simulink model "sampleModel1442"  (R2023a)
settings: Solver=VariableStepAuto  StartTime=0.0  StopTime=10.0  RelTol=1e-3
libraries: hdlsllib x5
settings Model: Creator=user1  LastModifiedBy=user1

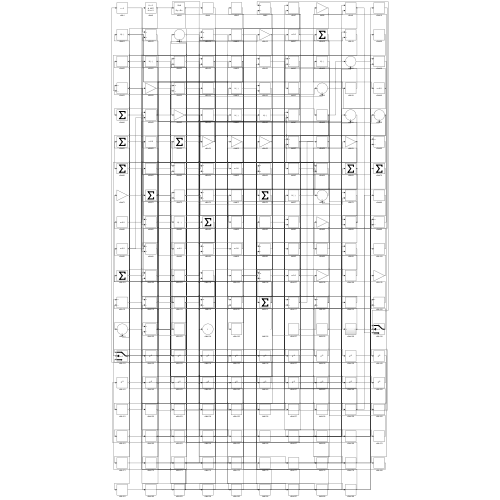
[thumbnail: Simulink's stored preview of the top-level diagram]
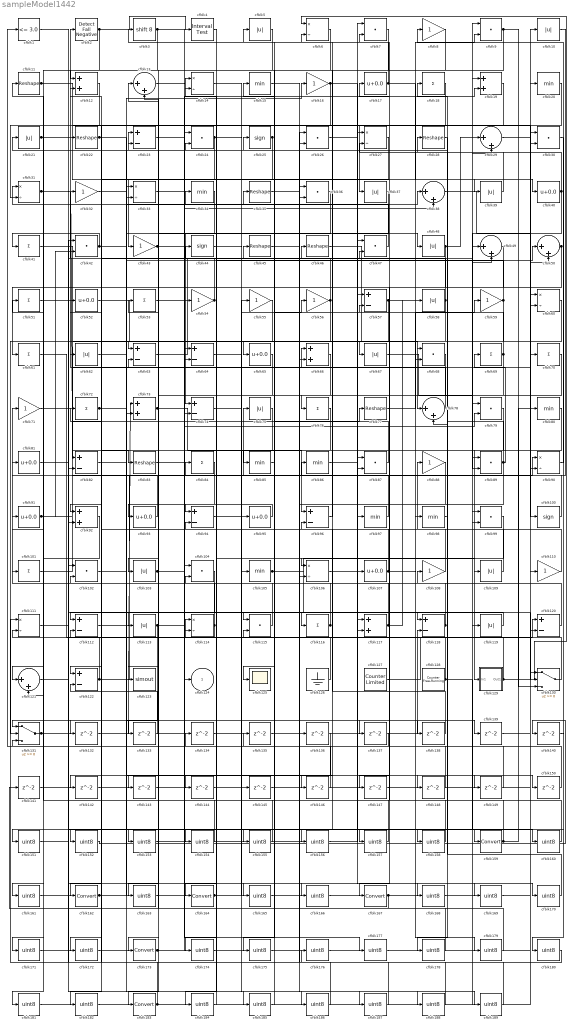
== system sampleModel1442 ==
  cfblk1 : hdlsllib/Logic and Bit Operations/Compare To Constant  relop=<=  const=3.0  OutDataTypeStr=boolean
  cfblk{5,10,21,37,39,48,58,62,67,75,103,109,113,119} (14 alike) : Abs  SaturateOnIntegerOverflow=off
  cfblk100 : Signum
  cfblk{18,41,51,53,61,69..70,72,76,84,101,116} (12 alike) : Sum  Inputs=+
  cfblk{7,9,24,26,30,36,42,47,68,79,87,89,99,102,104,115} (16 alike) : DotProduct  OutDataTypeStr=Inherit: Inherit via internal rule
  cfblk{15,20,34,80,85..86,97..98,105} (9 alike) : MinMax
  cfblk{6,14,27,31,33,60,90,106,111,114} (10 alike) : Product  Inputs=*/  RndMeth=Zero  SaturateOnIntegerOverflow=on
  cfblk{17,40,52,65,81,91,93,95,107} (9 alike) : Bias  Bias=0.0  SaturateOnIntegerOverflow=off
  cfblk{8,16,32,43,54..56,59,71,88,108,110} (12 alike) : Gain
  cfblk{11,22,28,35,45..46,77,83} (8 alike) : Reshape
  cfblk{23,57,63..64,74,82,94,96,112,118,120,122} (12 alike) : Sum  Inputs=+-
  cfblk{12,19,66,73,92,117} (6 alike) : Sum
  cfblk{13,29,38,49..50,78,121} (7 alike) : Sum  Inputs=|++
  cfblk123 : ToWorkspace  VariableName=simout  SaveFormat=Timeseries  SampleTime=-1
  cfblk125 : Scope
  cfblk126 : Ground
  cfblk127 : hdlsllib/Sources/Counter Limited  uplimit=7  tsamp=-1
  cfblk128 : hdlsllib/Sources/Counter Free-Running  NumBits=16  tsamp=-1
  cfblk129 : Subsystem
      settings: LibrarySourceBlock=|
      | hdlsllib/Ports &
      | Subsystems/Subsystem
  cfblk130 : Switch  SaturateOnIntegerOverflow=off  InputSameDT=off
  cfblk131 : Switch  SaturateOnIntegerOverflow=off  InputSameDT=off
  cfblk{132..150} (19 alike) : Delay  SampleTime=1
  cfblk{151..158,160..161,163,165..166,168..172,174..182,184..189} (33 alike) : DataTypeConversion  OutDataTypeStr=uint8  SaturateOnIntegerOverflow=off  RndMeth=Floor
  cfblk{159,162,164,167,173,183} (6 alike) : DataTypeConversion  SaturateOnIntegerOverflow=off  RndMeth=Floor
  cfblk2 : hdlsllib/Logic and Bit Operations/Detect Fall Negative  vinit=0  OutDataTypeStr=boolean
  cfblk25 : Signum
  cfblk3 : ArithShift  BitShiftNumber=8
  cfblk4 : hdlsllib/Logic and Bit Operations/Interval Test  IntervalClosedRight=on  uplimit=0.5  IntervalClosedLeft=on  lowlimit=-0.5  OutDataTypeStr=boolean
  cfblk44 : Signum
  cfblk124 : Outport  VectorParamsAs1DForOutWhenUnconnected=off
  wires:
  cfblk25/1 -> cfblk43/1, cfblk152/1
  cfblk59/1 -> cfblk63/1, cfblk14/1, cfblk131/2
  cfblk36/1 -> cfblk74/1
  cfblk90/1 -> cfblk8/1
  cfblk10/1 -> cfblk75/1
  cfblk87/1 -> cfblk112/1
  cfblk61/1 -> cfblk120/1
  cfblk101/1 -> cfblk77/1
  cfblk31/1 -> cfblk82/1, cfblk114/2
  cfblk107/1 -> cfblk35/1, cfblk169/1
  cfblk54/1 -> cfblk23/1, cfblk22/1
  cfblk79/1 -> cfblk129/1(In1)
  cfblk49/1 -> cfblk122/1
  cfblk129/1(Out1) -> cfblk6/1, cfblk53/1
  cfblk41/1 -> cfblk67/1
  cfblk47/1 -> cfblk31/1
  cfblk73/1 -> cfblk96/1, cfblk19/2
  cfblk55/1 -> cfblk162/1
  cfblk131/1 -> cfblk73/1, cfblk57/1
  cfblk50/1 -> cfblk61/1, cfblk174/1
  cfblk84/1 -> cfblk183/1
  cfblk99/1 -> cfblk164/1
  cfblk46/1 -> cfblk78/1
  cfblk51/1 -> cfblk83/1
  cfblk39/1 -> cfblk28/1
  cfblk56/1 -> cfblk12/2, cfblk171/1
  cfblk96/1 -> cfblk6/2
  cfblk6/1 -> cfblk65/1
  cfblk120/1 -> cfblk18/1
  cfblk105/1 -> cfblk109/1, cfblk130/2
  cfblk37/1 -> cfblk116/1
  cfblk63/1 -> cfblk46/1
  cfblk85/1 -> cfblk25/1
  cfblk78/1 -> cfblk2/1
  cfblk122/1 -> cfblk90/1, cfblk52/1, cfblk91/1, cfblk150/1, cfblk158/1
  cfblk72/1 -> cfblk16/1, cfblk149/1
  cfblk76/1 -> cfblk123/1
  cfblk115/1 -> cfblk32/1
  cfblk112/1 -> cfblk118/1
  cfblk109/1 -> cfblk88/1
  cfblk108/1 -> cfblk62/1
  cfblk93/1 -> cfblk51/1
  cfblk89/1 -> cfblk21/1, cfblk69/1, cfblk106/2
  cfblk81/1 -> cfblk47/2
  cfblk38/1 -> cfblk100/1
  cfblk83/1 -> cfblk66/1
  cfblk11/1 -> cfblk97/1, cfblk90/2
  cfblk97/1 -> cfblk86/1
  cfblk114/1 -> cfblk11/1, cfblk111/2
  cfblk100/1 -> cfblk23/2
  cfblk69/1 -> cfblk45/1, cfblk143/1, cfblk144/1
  cfblk126/1 -> cfblk63/2
  cfblk9/1 -> cfblk85/1, cfblk130/3
  cfblk24/1 -> cfblk95/1, cfblk92/1
  cfblk88/1 -> cfblk106/1
  cfblk127/1 -> cfblk79/1
  cfblk128/1 -> cfblk57/2, cfblk160/1
  cfblk12/1 -> cfblk31/2
  cfblk98/1 -> cfblk78/2
  cfblk16/1 -> cfblk121/1, cfblk40/1
  cfblk2/1 -> cfblk4/1, cfblk12/1
  cfblk95/1 -> cfblk93/1
  cfblk103/1 -> cfblk24/1, cfblk38/2
  cfblk60/1 -> cfblk167/1
  cfblk52/1 -> cfblk98/1
  cfblk67/1 -> cfblk89/1
  cfblk18/1 -> cfblk37/1
  cfblk3/1 -> cfblk68/1, cfblk131/1
  cfblk22/1 -> cfblk48/1, cfblk182/1
  cfblk66/1 -> cfblk94/1
  cfblk34/1 -> cfblk173/1
  cfblk118/1 -> cfblk113/1, cfblk101/1
  cfblk4/1 -> cfblk64/1
  cfblk130/1 -> cfblk114/1
  cfblk113/1 -> cfblk79/2, cfblk161/1
  cfblk29/1 -> cfblk20/1
  cfblk14/1 -> cfblk68/2
  cfblk19/1 -> cfblk82/2
  cfblk77/1 -> cfblk59/1
  cfblk116/1 -> cfblk71/1, cfblk5/1
  cfblk42/1 -> cfblk41/1, cfblk38/1
  cfblk71/1 -> cfblk10/1
  cfblk110/1 -> cfblk44/1
  cfblk40/1 -> cfblk89/2, cfblk27/2
  cfblk33/1 -> cfblk159/1
  cfblk21/1 -> cfblk105/1, cfblk121/2
  cfblk17/1 -> cfblk3/1, cfblk39/1
  cfblk58/1 -> cfblk74/2, cfblk14/2
  cfblk119/1 -> cfblk115/1
  cfblk48/1 -> cfblk29/1, cfblk146/1, cfblk147/1
  cfblk65/1 -> cfblk103/1
  cfblk91/1 -> cfblk64/2, cfblk42/2
  cfblk106/1 -> cfblk107/1
  cfblk117/1 -> cfblk72/1, cfblk58/1
  cfblk94/1 -> cfblk56/1
  cfblk80/1 -> cfblk125/1
  cfblk62/1 -> cfblk50/1
  cfblk68/1 -> cfblk76/1
  cfblk43/1 -> cfblk139/1, cfblk157/1
  cfblk57/1 -> cfblk9/2, cfblk92/2, cfblk179/1
  cfblk53/1 -> cfblk19/1
  cfblk64/1 -> cfblk117/2
  cfblk75/1 -> cfblk132/1
  cfblk132/1 -> cfblk118/2
  cfblk8/1 -> cfblk133/1
  cfblk133/1 -> cfblk122/2
  cfblk134/1 -> cfblk87/1
  cfblk135/1 -> cfblk36/2
  cfblk35/1 -> cfblk136/1
  cfblk82/1 -> cfblk137/1
  cfblk137/1 -> cfblk1/1
  cfblk86/1 -> cfblk138/1
  cfblk138/1 -> cfblk96/2
  cfblk139/1 -> cfblk120/2
  cfblk141/1 -> cfblk49/2
  cfblk20/1 -> cfblk142/1
  cfblk142/1 -> cfblk73/2
  cfblk143/1 -> cfblk66/2
  cfblk144/1 -> cfblk94/2
  cfblk145/1 -> cfblk117/1
  cfblk146/1 -> cfblk24/2
  cfblk147/1 -> cfblk50/2
  cfblk32/1 -> cfblk148/1
  cfblk148/1 -> cfblk27/1
  cfblk149/1 -> cfblk112/2
  cfblk150/1 -> cfblk131/3
  cfblk140/1 -> cfblk151/1
  cfblk152/1 -> cfblk140/1
  cfblk104/1 -> cfblk153/1
  cfblk153/1 -> cfblk87/2
  cfblk1/1 -> cfblk154/1
  cfblk154/1 -> cfblk104/1
  cfblk151/1 -> cfblk155/1
  cfblk155/1 -> cfblk104/2
  cfblk7/1 -> cfblk156/1
  cfblk156/1 -> cfblk47/1
  cfblk157/1 -> cfblk7/1
  cfblk158/1 -> cfblk7/2
  cfblk159/1 -> cfblk81/1, cfblk80/1, cfblk17/1
  cfblk160/1 -> cfblk33/1
  cfblk161/1 -> cfblk33/2
  cfblk162/1 -> cfblk145/1, cfblk54/1
  cfblk27/1 -> cfblk163/1
  cfblk163/1 -> cfblk55/1
  cfblk164/1 -> cfblk134/1, cfblk110/1
  cfblk23/1 -> cfblk165/1
  cfblk165/1 -> cfblk99/1
  cfblk121/1 -> cfblk166/1
  cfblk166/1 -> cfblk99/2
  cfblk167/1 -> cfblk141/1, cfblk29/2, cfblk9/1
  cfblk45/1 -> cfblk168/1
  cfblk168/1 -> cfblk60/1
  cfblk169/1 -> cfblk60/2
  cfblk26/1 -> cfblk170/1
  cfblk170/1 -> cfblk108/1
  cfblk171/1 -> cfblk26/1
  cfblk136/1 -> cfblk172/1
  cfblk172/1 -> cfblk26/2
  cfblk173/1 -> cfblk124/1, cfblk130/1
  cfblk174/1 -> cfblk34/1
  cfblk70/1 -> cfblk175/1
  cfblk175/1 -> cfblk115/2
  cfblk176/1 -> cfblk70/1
  cfblk13/1 -> cfblk177/1
  cfblk177/1 -> cfblk119/1
  cfblk28/1 -> cfblk178/1
  cfblk178/1 -> cfblk13/1
  cfblk179/1 -> cfblk13/2
  cfblk30/1 -> cfblk180/1
  cfblk180/1 -> cfblk176/1
  cfblk92/1 -> cfblk181/1
  cfblk181/1 -> cfblk30/1
  cfblk182/1 -> cfblk30/2
  cfblk183/1 -> cfblk111/1, cfblk42/1, cfblk49/1
  cfblk5/1 -> cfblk184/1
  cfblk184/1 -> cfblk84/1
  cfblk102/1 -> cfblk185/1
  cfblk185/1 -> cfblk135/1
  cfblk111/1 -> cfblk186/1
  cfblk186/1 -> cfblk102/1
  cfblk74/1 -> cfblk187/1
  cfblk187/1 -> cfblk102/2
  cfblk15/1 -> cfblk188/1
  cfblk188/1 -> cfblk36/1
  cfblk44/1 -> cfblk189/1
  cfblk189/1 -> cfblk15/1

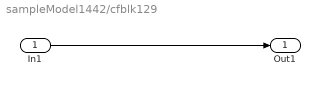
== system sampleModel1442/cfblk129 ==
  In1 : Inport
  Out1 : Outport
  wires:
  In1/1 -> Out1/1
